simulink model "lipm"  (R2020b)
settings: Solver=ode4  StartTime=0.0  StopTime=t_stop  RelTol=1e-3
values from neighbouring files (symbols this model uses):
  tao_x = 0    [data_file.m]    (also in graph_zmp.m = ans(5,:); mf2_zmp.m = u(1))
  tao_y = 0    [data_file.m]    (also in graph_zmp.m = ans(9,:); mf3_zmp.m = u(1))
  zc = 1.54    [data.m]    (also in data_file.m = 0.154; graph_file.m = ans(4,:); graph_zmp.m = ans(10,:))
settings Model: Creator=Vedang  LastModifiedBy=Vedang
settings DebuggingCC: UnconnectedInputMsg=none  UnconnectedOutputMsg=none  UnconnectedLineMsg=none
settings ModelReferenceCC: EnableRefExpFcnMdlSchedulingChecks=off

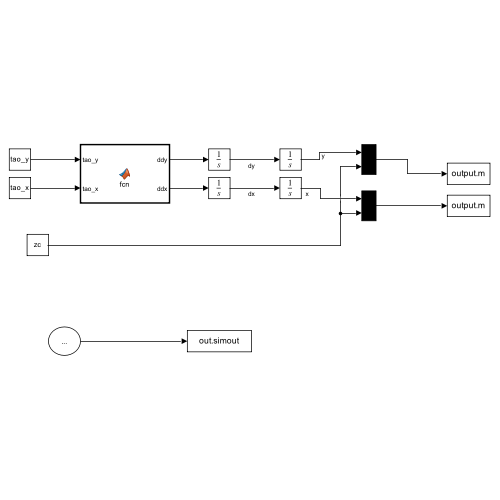
[thumbnail: Simulink's stored preview of the top-level diagram]
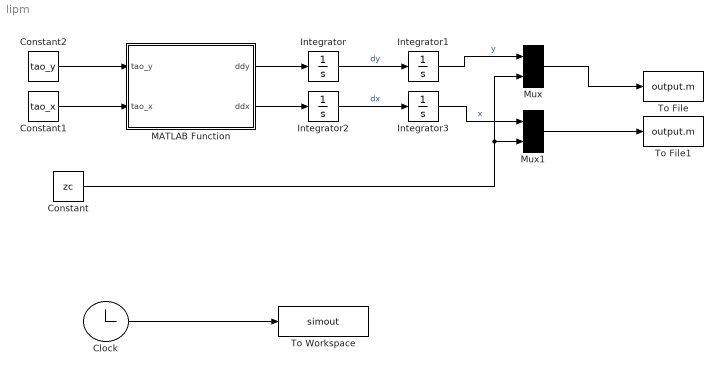
== system lipm ==
  Clock : Clock
  Constant : Constant  Value=zc
  Constant1 : Constant  Value=tao_x
  Constant2 : Constant  Value=tao_y
  Integrator{,1..3} (4 alike) : Integrator
  MATLAB Function : MATLAB Function  TreatAsAtomicUnit=on
  Mux : Mux  Inputs=2
  Mux1 : Mux  Inputs=2
  To File : ToFile  Filename=output.m  SaveFormat=Timeseries
  To File1 : ToFile  Filename=output.m  SaveFormat=Timeseries
  To Workspace : ToWorkspace  VariableName=simout  SaveFormat=Timeseries  SampleTime=-1
  wires:
  MATLAB Function/1(ddy) -> Integrator/1
  Integrator/1 -> Integrator1/1  "dy"
  MATLAB Function/2(ddx) -> Integrator2/1
  Integrator2/1 -> Integrator3/1  "dx"
  Integrator1/1 -> Mux/1  "y"
  Mux/1 -> To File/1
  Constant/1 -> Mux1/2, Mux/2
  Integrator3/1 -> Mux1/1  "x"
  Mux1/1 -> To File1/1
  Constant1/1 -> MATLAB Function/2(tao_x)
  Constant2/1 -> MATLAB Function/1(tao_y)
  Clock/1 -> To Workspace/1

== matlab function lipm/MATLAB Function ==
  data: tao_y input; tao_x input; ddy output; ddx output
function [ddy,ddx] = fcn(tao_y,tao_x)
ddy= ((g/zc)*y - (1/(m*zc))*tao_y);
ddx= ((g/zc)*x + (1/(m*zc))*tao_x);
